simulink model "Simulink_Model_Konfiguration_Q_z"  (R2022b)
settings: Solver=FixedStepAuto  StartTime=0.0  StopTime=t_control_loop_end + 3600*4  FixedStep=0.5  RelTol=1e-3
values from neighbouring files (symbols this model uses):
  c = par.c    [Iteration_1.m]    (also in SIMULATION_EXPERIMENT_18.m; SIMULATION_EXPERIMENT_18_14Parameter.m; Summary_Results_Plots.m = door_color)
  th_tot = theta_vektor.*f_1    [Summary_Results_Plots.m]
undefined symbols (not defined in the file or in its folder): door_closed, door_open, Ki_control_tune, Kp_control_tune, T_desired
settings Model: Creator=yanni  LastModifiedBy=yanni
settings DebuggingCC: UnconnectedInputMsg=warning  UnconnectedOutputMsg=warning  UnconnectedLineMsg=warning
settings ModelReferenceCC: EnableRefExpFcnMdlSchedulingChecks=on
settings RTWCC: DLArmComputeVersion=19.05

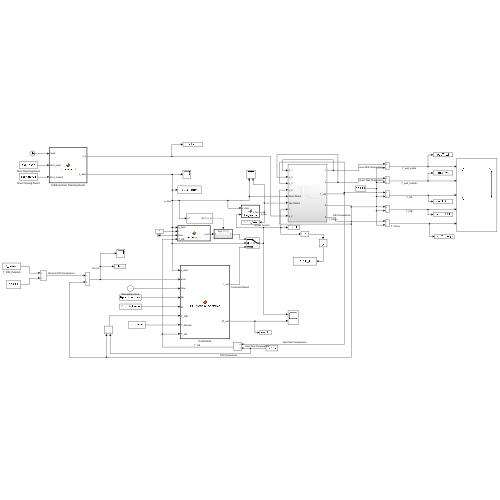
[thumbnail: Simulink's stored preview of the top-level diagram]
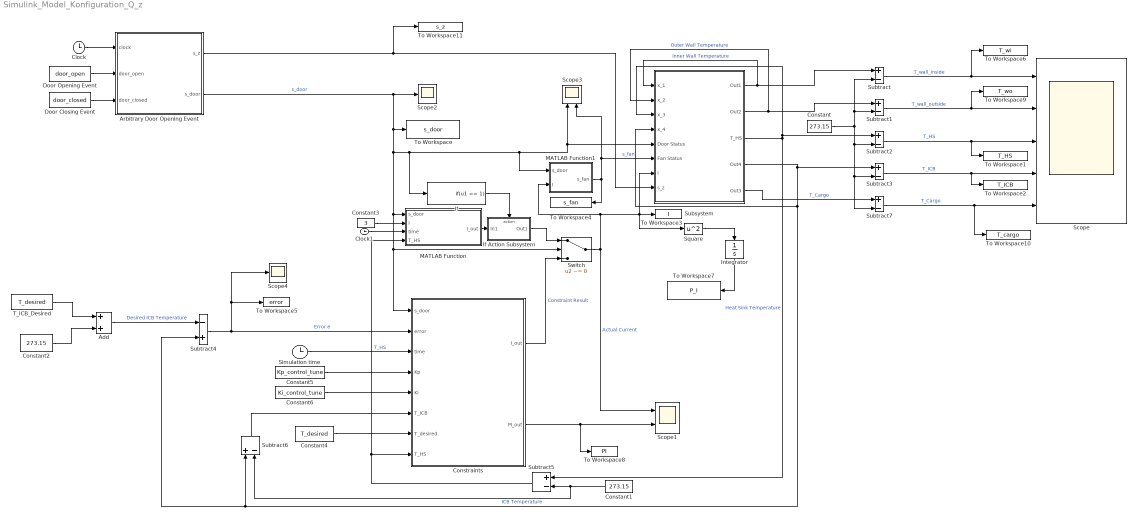
== system Simulink_Model_Konfiguration_Q_z ==
  Add : Sum
  Arbitrary Door Opening Event : MATLAB Function  TreatAsAtomicUnit=on
  Clock : Clock
  Clock1 : Clock
  Constant : Constant  Value=273.15
  Constant1 : Constant  Value=273.15
  Constant2 : Constant  Value=273.15
  Constant3 : Constant  Value=3
  Constant4 : Constant  Value=T_desired
  Constant5 : Constant  Value=Kp_control_tune
  Constant6 : Constant  Value=Ki_control_tune
  Constraints : MATLAB Function  TreatAsAtomicUnit=on
  Door Closing Event : Constant  Value=door_closed
  Door Opening Event : Constant  Value=door_open
  If : If  IfExpression=u1 == 1  ShowElse=off
  If Action Subsystem : Subsystem  TreatAsAtomicUnit=on
  Integrator : Integrator
  MATLAB Function : MATLAB Function  TreatAsAtomicUnit=on
  MATLAB Function1 : MATLAB Function  TreatAsAtomicUnit=on
  Scope : Scope  NumInputPorts=5
  Scope1 : Scope  NumInputPorts=2
  Scope2 : Scope
  Scope3 : Scope  NumInputPorts=2
  Scope4 : Scope
  Simulation time : Clock
  Square : Math  Operator=square
  Subsystem : Subsystem
  Subtract{,1..3,5..7} (7 alike) : Sum  Inputs=+-
  Subtract4 : Sum  Inputs=-+
  Switch : Switch  Criteria=u2 ~= 0  SaturateOnIntegerOverflow=off  InputSameDT=off
  T_ICB_Desired : Constant  Value=T_desired
  To Workspace : ToWorkspace  VariableName=s_door  SaveFormat=Timeseries  SampleTime=-1
  To Workspace1 : ToWorkspace  VariableName=T_HS  SaveFormat=Timeseries  SampleTime=-1
  To Workspace10 : ToWorkspace  VariableName=T_cargo  SaveFormat=Timeseries  SampleTime=-1
  To Workspace11 : ToWorkspace  VariableName=s_z  SaveFormat=Timeseries  SampleTime=-1
  To Workspace2 : ToWorkspace  VariableName=T_ICB  SaveFormat=Timeseries  SampleTime=-1
  To Workspace3 : ToWorkspace  VariableName=I  SaveFormat=Timeseries  SampleTime=-1
  To Workspace4 : ToWorkspace  VariableName=s_fan  SaveFormat=Timeseries  SampleTime=-1
  To Workspace5 : ToWorkspace  VariableName=error  SaveFormat=Timeseries  SampleTime=-1
  To Workspace6 : ToWorkspace  VariableName=T_wi  SaveFormat=Timeseries  SampleTime=-1
  To Workspace7 : ToWorkspace  VariableName=P_I  SaveFormat=Timeseries  SampleTime=-1
  To Workspace8 : ToWorkspace  VariableName=PI  SaveFormat=Timeseries  SampleTime=-1
  To Workspace9 : ToWorkspace  VariableName=T_wo  SaveFormat=Timeseries  SampleTime=-1
  wires:
  Subsystem/1(Out1) -> Subtract/1, Subsystem/1(x_1)  "Inner Wall Temperature"
  Subsystem/2(Out2) -> Subtract1/1, Subsystem/2(x_2)  "Outer Wall Temperature"
  Subsystem/3(T_HS) -> Subsystem/3(x_3), Subtract2/1, Subtract5/1  "Heat Sink Temperature"
  Subsystem/4(Out4) -> Subtract6/1, Subtract4/2, Subsystem/4(x_4), Subtract3/1  "ICB Temperature"
  Constant/1 -> Subtract7/2, Subtract3/2, Subtract2/2, Subtract1/2, Subtract/2
  Subtract/1 -> To Workspace6/1, Scope/1  "T_wall_inside"
  Subtract1/1 -> To Workspace9/1, Scope/2  "T_wall_outside"
  Subtract2/1 -> To Workspace1/1, Scope/3  "T_HS"
  Subtract3/1 -> To Workspace2/1, Scope/4  "T_ICB"
  T_ICB_Desired/1 -> Add/1
  Constant2/1 -> Add/2
  Add/1 -> Subtract4/1  "Desired ICB Temperature"
  Subtract4/1 -> Scope4/1, To Workspace5/1, Constraints/2(error)  "Error e"
  MATLAB Function1/1(s_fan) -> Subsystem/6(Fan Status), Scope3/2, To Workspace4/1  "s_fan"
  Clock/1 -> Arbitrary Door Opening Event/1(clock)
  Door Closing Event/1 -> Arbitrary Door Opening Event/3(door_closed)
  Door Opening Event/1 -> Arbitrary Door Opening Event/2(door_open)
  Arbitrary Door Opening Event/2(s_door) -> To Workspace/1, If/1, Scope3/1, Subsystem/5(Door Status), MATLAB Function1/1(s_door), Constraints/1(s_door), Switch/2, MATLAB Function/1(s_door), Scope2/1  "s_door"
  If/1 -> If Action Subsystem/Action
  Constant3/1 -> MATLAB Function/2(I)
  If Action Subsystem/1(Out1) -> Switch/1
  Switch/1 -> Scope1/1, Square/1, Subsystem/7(I), To Workspace3/1, MATLAB Function1/2(I)  "Actual Current"
  Constraints/1(I_out) -> Switch/3  "Constraint Result"
  Simulation time/1 -> Constraints/3(time)
  Constant1/1 -> Subtract6/2, Subtract5/2
  Subtract5/1 -> MATLAB Function/4(T_HS), Constraints/8(T_HS)  "T_HS"
  Subtract6/1 -> Constraints/6(T_ICB)
  Constant4/1 -> Constraints/7(T_desired)
  Square/1 -> Integrator/1
  Integrator/1 -> To Workspace7/1
  Constant5/1 -> Constraints/4(Kp)
  Constant6/1 -> Constraints/5(Ki)
  Constraints/2(PI_out) -> Scope1/2, To Workspace8/1
  MATLAB Function/1(I_out) -> If Action Subsystem/1(In1)
  Clock1/1 -> MATLAB Function/3(time)
  Arbitrary Door Opening Event/1(s_z) -> To Workspace11/1, Subsystem/8(s_z)
  Subsystem/5(Out3) -> Subtract7/1  "T_Cargo"
  Subtract7/1 -> To Workspace10/1, Scope/5  "T_Cargo"

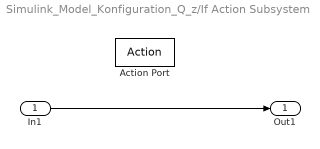
== system Simulink_Model_Konfiguration_Q_z/If Action Subsystem ==
  In1 : Inport
  Action Port : ActionPort  ActionPortLabel=if(u1 == 1)
  Out1 : Outport
  wires:
  In1/1 -> Out1/1

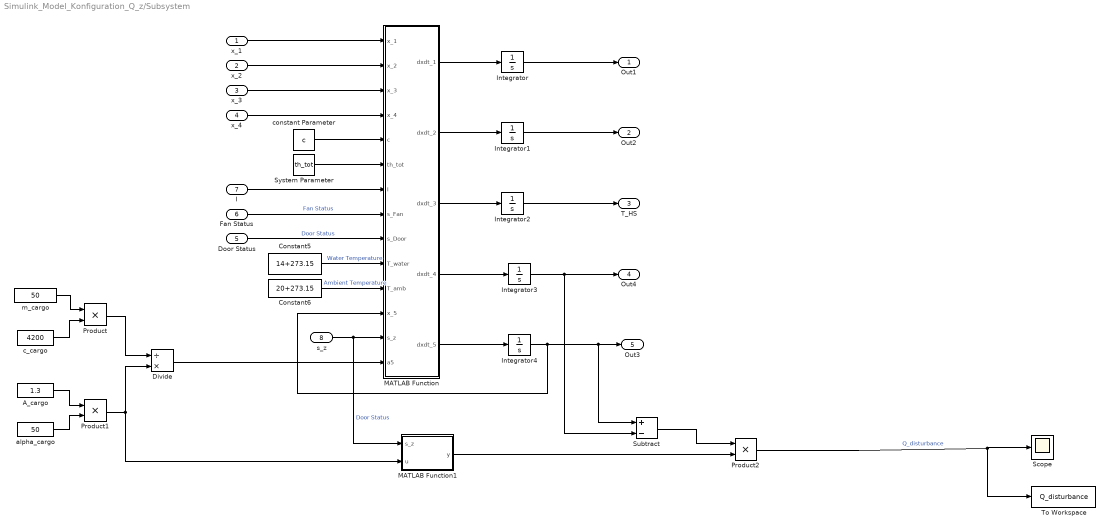
== system Simulink_Model_Konfiguration_Q_z/Subsystem ==
  x_1 : Inport
  x_2 : Inport  Port=2
  x_3 : Inport  Port=3
  x_4 : Inport  Port=4
  Door Status : Inport  Port=5
  Fan Status : Inport  Port=6
  I : Inport  Port=7
  s_z : Inport  Port=8
  A_cargo : Constant  Value=1.3
  Constant5 : Constant  Value=14+273.15
  Constant6 : Constant  Value=20+273.15
  Divide : Product  Inputs=/*
  Integrator{,1..4} (5 alike) : Integrator  InitialCondition=20+273.15
  MATLAB Function : MATLAB Function  TreatAsAtomicUnit=on
  MATLAB Function1 : MATLAB Function  TreatAsAtomicUnit=on
  Product : Product
  Product1 : Product
  Product2 : Product
  Scope : Scope
  Subtract : Sum  Inputs=+-
  System Parameter : Constant  Value=th_tot
  To Workspace : ToWorkspace  VariableName=Q_disturbance  SaveFormat=Timeseries  SampleTime=-1
  alpha_cargo : Constant  Value=50
  c_cargo : Constant  Value=4200
  constant Parameter : Constant  Value=c
  m_cargo : Constant  Value=50
  Out1 : Outport
  Out2 : Outport  Port=2
  T_HS : Outport  Port=3
  Out4 : Outport  Port=4
  Out3 : Outport  Port=5
  wires:
  MATLAB Function/3(dxdt_3) -> Integrator2/1
  x_2/1 -> MATLAB Function/2(x_2)
  Integrator/1 -> Out1/1
  Integrator1/1 -> Out2/1
  Integrator2/1 -> T_HS/1
  MATLAB Function/1(dxdt_1) -> Integrator/1
  System Parameter/1 -> MATLAB Function/6(th_tot)
  MATLAB Function/4(dxdt_4) -> Integrator3/1
  x_3/1 -> MATLAB Function/3(x_3)
  x_1/1 -> MATLAB Function/1(x_1)
  Door Status/1 -> MATLAB Function/9(s_Door)  "Door Status"
  I/1 -> MATLAB Function/7(I)
  Constant5/1 -> MATLAB Function/10(T_water)  "Water Temperature"
  Constant6/1 -> MATLAB Function/11(T_amb)  "Ambient Temperature"
  Integrator3/1 -> Subtract/2, Out4/1
  Fan Status/1 -> MATLAB Function/8(s_Fan)  "Fan Status"
  constant Parameter/1 -> MATLAB Function/5(c)
  MATLAB Function/2(dxdt_2) -> Integrator1/1
  x_4/1 -> MATLAB Function/4(x_4)
  MATLAB Function/5(dxdt_5) -> Integrator4/1
  Integrator4/1 -> Subtract/1, Out3/1, MATLAB Function/12(x_5)
  s_z/1 -> MATLAB Function1/1(s_z), MATLAB Function/13(s_z)  "Door Status"
  Divide/1 -> MATLAB Function/14(a5)
  m_cargo/1 -> Product/1
  c_cargo/1 -> Product/2
  A_cargo/1 -> Product1/1
  alpha_cargo/1 -> Product1/2
  Product1/1 -> MATLAB Function1/2(u), Divide/2
  Product/1 -> Divide/1
  Product2/1 -> To Workspace/1, Scope/1  "Q_disturbance"
  MATLAB Function1/1(y) -> Product2/2
  Subtract/1 -> Product2/1

== matlab function Simulink_Model_Konfiguration_Q_z/Arbitrary Door Opening Event ==
  data: s_z output; clock input; door_open input; s_door output; door_closed input
function [s_z, s_door] = door_control(clock, door_open, door_closed)
    % Determine the current time in the simulation
    t = clock;
    s_door = 0;

    if t >= door_open(1)
        idx = 1;
        while_cond = true;
        while while_cond == true && idx < (numel(door_open)+1)
            if t >= door_open(idx) && t <= door_closed(idx)
                s_door = 1;
                while_cond = false;
            else
                if idx <= numel(door_open)
                    idx = idx +1;
                    s_door = 0;
                else
                    s_door = 0;
                    while_cond = false;
                end
            end
        end
    else
        s_door = 0;
    end
    
    % Set value for Q_disturbance:
    if t >= door_closed(end)
        s_z = 1; % 1
    else
        s_z = 0;
    end
end

== matlab function Simulink_Model_Konfiguration_Q_z/Subsystem/MATLAB Function ==
  data: x_1 input; dxdt_1 output; x_2 input; x_3 input; x_4 input; c input; th_tot input; I input; s_Fan input; s_Door input; T_water input; T_amb input; dxdt_2 output; dxdt_3 output; dxdt_4 output; x_5 input; s_z input; a5 input; dxdt_5 output
function [dxdt_1, dxdt_2, dxdt_3, dxdt_4, dxdt_5] = ICB(x_1,x_2,x_3,x_4,c,...
    th_tot,I,s_Fan,s_Door,T_water,T_amb, x_5, s_z, a5)

th = th_tot;
x = [x_1, x_2, x_3, x_4, x_5];


%%%%%%%%%%%%%%%%%%%%%%%%%%%%%%%%%%%%%%%%%%%%%%%%%%%%%%%%%%%%%%%%%%%%%%%%%%%
% Data_18 = par.Data;
% t_Data = Data_18(:,1);
% 
% s_Door_ref = Data_18(:,7);
% s_Door = interp1(t_Data, s_Door_ref, t, 'previous');
% 
% I_ref = Data_18(:,6);
% I = interp1(t_Data, I_ref, t, 'previous');
% 
% s_Fan_ref = Data_18(:,8);
% s_Fan = interp1(t_Data, s_Fan_ref, t, 'previous');
% 
% T_water_ref = Data_18(:,4)+273.15;
% T_water = interp1(t_Data, T_water_ref, t, 'previous');
% 
% T_amb_ref = Data_18(:,5)+273.15;
% T_amb = interp1(t_Data, T_amb_ref, t, 'previous');

%%%%%%%%%%%%%%%%%%%%%%%%%%%%%%%%%%%%%%%%%%%%%%%%%%%%%%%%%%%%%%%%%%%%%%%%%%%


%Beschreibung des Vektors x:
% x(1) -> T_wall_inside
% x(2) -> T_wall_outside
% x(3) -> T_cargo
% x(4) -> T_hs
% x(5) -> T_ICB
% x(6) -> (V_punkt / A_ap) [m/s]


%All 6 Differential Equations
dxdt_1 = th(1)*(x(2)-x(1)) - th(2)*(x(1)-x(4));
dxdt_2 = th(3)*(T_amb-x(2)) - c(2)*(x(2)-x(1));
dxdt_3 = (th(4)*s_Fan + (1-s_Fan)*th(5))*(x(4)-x(3)) -...
    th(6)*I*x(3) + ...
    th(7)*(I^2) +...
    th(8)*(T_water-x(3));
dxdt_4 = th(9)*(x(1)-x(4)) - ...
    (th(10)*s_Fan + (1-s_Fan)*th(11))*(x(4)-x(3)) + ...
    th(12)*(T_amb-x(4))*s_Door +...
    th(13)*s_Fan + s_z*a5*(x_5-x_4);
dxdt_5 = -s_z*a5*(x_5-x_4);

end

== matlab function Simulink_Model_Konfiguration_Q_z/MATLAB Function1 ==
  data: s_door input; s_fan output; I input
function s_fan = fan_status(s_door, I)

    if s_door == 1
        s_fan = 0;
    else % s_door == 0 (closed)
        if I == 0
            s_fan = 0;
        else
            s_fan = 1;
        end
    end

end

== matlab function Simulink_Model_Konfiguration_Q_z/Constraints ==
  settings: updateMethod=DISCRETE
  data: s_door input; error input; I_out output; time input; Kp input; Ki input; T_ICB input; T_desired input; T_HS input; PI_out output
function [I_out, PI_out] = PI_Hysteresis_Controller(s_door, error, time, Kp, Ki, ...
    T_ICB, T_desired, T_HS)

persistent clock state prev_PI prev_door prev_error

% Set initial values
I_out = NaN;
if isempty(state) || isempty(clock)
    if error > 0
        state = 'on';
    else
        state = 'off'; % Compressor is initially off
    end
    clock = 0; % Start Clock
    prev_door = s_door;
    prev_error = error; % Ghost Point is set to the current error!
    prev_PI = 0; % Initalize PI at t = 0
end

% Check if Door changes!
% if (prev_door == 0) && (s_door == 1)
%     prev_PI = 0;
% end
% prev_door = s_door; % Update previous door status!

PI_out = prev_PI + Kp*error + (Ki*0.5 - Kp)*prev_error;

if PI_out < 0
    PI_out = 0;
elseif PI_out > 7
    PI_out = 7;
end

% Update error and the PI value:
prev_error = error;
prev_PI = PI_out;


e = T_ICB - T_desired;

if strcmp(state,'off') % Compressor is currently off
    if e < 0.3
        I_out = 0;
    elseif (e >= 0.3) && ((time-clock) < 100)
        I_out = 0;
    elseif (e >= 0.3) && ((time-clock)>= 100)
        if PI_out >= 3
            I_out = PI_out;
        else
            I_out = 3;
        end
        state = 'on';
        clock = time;
    end

else % Compressor is currently on!
    if T_HS <= -10
        I_out = 0;
        state = 'off';
        clock = time;
    else % T_HS > -10
        if e >= -0.5
            if PI_out >= 3
                I_out = PI_out;
            else
                I_out = 3;
            end
        else
            I_out = 0;
            state = 'off';
            clock = time;
            prev_PI = 0; % Added
        end
    end
end


end

== matlab function Simulink_Model_Konfiguration_Q_z/MATLAB Function ==
  settings: updateMethod=DISCRETE
  data: s_door input; I input; I_out output; time input; T_HS input
function I_out = logic_operator(s_door, I, time, T_HS)

persistent clock state I_actual

% Set initial values
I_out = NaN;
if isempty(state) || isempty(clock)
    if s_door == 1
        state = 'on';
        I_actual = I;
    else
        state = 'off';
        I_actual = 0;
    end
    clock = 0; % Start Clock
end



if strcmp(state, 'on')
    if s_door == 1 % Door is open
        if T_HS > -10
            I_actual = I;
        else
            I_actual = 0;
            state = 'off';
            clock = time;
        end
    else % Door is closed
        state = 'off';
        I_actual = 0;
        clock = time;
    end
else % Peltier Element is off:
    if s_door == 0 % Door is closed
        I_actual = 0;
    else % Door is open
        if T_HS <= -10
            I_actual = 0;
        else
            if (time-clock) < 100
                I_actual = 0;
            else
                I_actual = I;
                state = 'on';
                clock = time;
            end
        end
    end
end

I_out = I_actual;

== matlab function Simulink_Model_Konfiguration_Q_z/Subsystem/MATLAB Function1 ==
  data: s_z input; u input; y output
function y = fcn(s_z, u)

if s_z == 0
    y = 0;
else
    y = u;
end
